simulink model "Two_Zone_MVDC_PSolver_Thermal"  (R2025b)
settings: Solver=FixedStepDiscrete  StartTime=0.0  StopTime=30  FixedStep=TsELEC  RelTol=1e-3  EnableMultiTasking=on
InitFcn:
  | TsELEC = 25e-6;
  | Ts = 25e-6;
  | TsTHERMAL = 1e-3;
  | TsCont = TsELEC;
  | Rsnub = 1e4;
undefined symbols (not defined in the file or in its folder): DiscIntNeverNeededParam, ee_sli_rtmsupport, GABDA, GABDB, GBBDA, GBBDB, gcbh, GPMMA, GPPMB, GPPMC, SADA, SADB, SADC, SADD, SBDA, SBDB, SBDC, SCDA, SCDB, SCDC, SCDD, SDDA, SDDB, SDDC, SDDD, SDDE
libraries: fl_lib x182, nesl_utility x93, ee_lib x50, SimscapeFluids_lib x4, simulink x3, slpidlib x3, eeSmAC1C x2, eePowerMeasurement x2, mcbeeMathTransformLib x2, eeTransforms x1
(part 4 of 5)

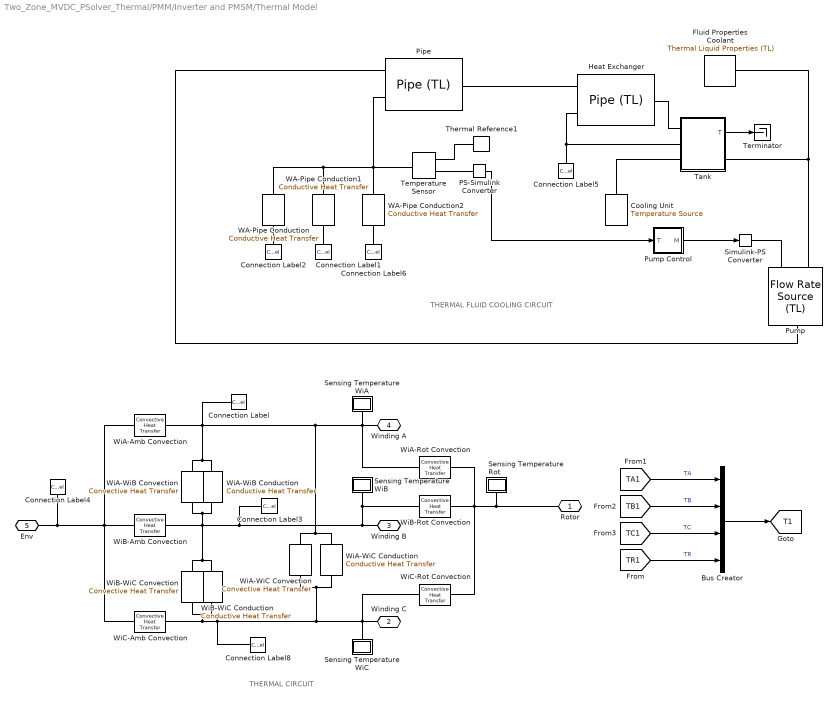
== system Two_Zone_MVDC_PSolver_Thermal/PMM/Inverter and PMSM/Thermal Model ==
  note: THERMAL CIRCUIT
  note: THERMAL FLUID COOLING CIRCUIT
  Bus Creator : BusCreator  Inputs=4
  Connection Label : ConnectionLabel  Label=WindingA
  Connection Label1 : ConnectionLabel  Label=WindingB
  Connection Label2 : ConnectionLabel  Label=WindingA
  Connection Label3 : ConnectionLabel  Label=WindingB
  Connection Label4 : ConnectionLabel  Label=Env
  Connection Label5 : ConnectionLabel  Label=Env
  Connection Label6 : ConnectionLabel  Label=WindingC
  Connection Label8 : ConnectionLabel  Label=WindingC
  Cooling Unit : fl_lib/Thermal/Thermal Sources/Temperature Source  temperature=278 K
  "Fluid Properties Coolant " : SimscapeFluids_lib/Thermal Liquid/Utilities/Thermal Liquid Properties (TL)  fluid_list=fluids.thermal_liquid.utilities.enum.thermal_liquid_fluid_list.ethylene_glycol  concentration_param_EG=fluids.thermal_liquid.utilities.enum.thermal_liquid_concentration.volume_fraction  concentration_param_PG=fluids.thermal_liquid.utilities.enum.thermal_liquid_concentration.volume_fraction  c_mass_SW=3.5e-3  c_mass_EG=0.1  c_mass_PG=0.1  c_mass_GL=0.1  c_vol_EG=0.1  c_vol_PG=0.1  beta_const_EG=2.1791 GPa  beta_const_PG=2.1791 GPa  beta_const_GL=2.1791 GPa  p_min_EG=0.01 MPa  p_min_PG=0.01 MPa  p_min_GL=0.01 MPa  p_max_EG=50 MPa  p_max_PG=50 MPa  p_max_GL=50 MPa  p_atm=0.101325 MPa  properties_range_check=simscape.enum.assert.action.error
  Heat Exchanger : SimscapeFluids_lib/Thermal Liquid/Pipes & Fittings/Pipe (TL)  dynamic_compressibility=0  inertia=0  num_segments=1  pipe_length=10 m  cross_section_geometry=fluids.thermal_liquid.pipes_fittings.enum.CrossSectionGeometry.Custom  pipe_diameter=0.1 m  pipe_inner_diameter=0.05 m  pipe_outer_diameter=0.1 m  pipe_width=0.1 m  pipe_height=0.1 m  pipe_major_axis=0.1 m  pipe_minor_axis=0.05 m  pipe_side=0.1 m  pipe_angle=30 deg  area=0.1^2/4*pi m^2  Dh=0.1128 m  elevation_spec=foundation.enum.constant_variable.constant  elevation_gain=0 m  gravity_spec=foundation.enum.constant_variable.constant  g=9.81 m/s^2  pressure_loss_spec=1  local_pressure_loss_spec=fluids.thermal_liquid.pipes_fittings.enum.LocalLossSpec.AggregateLength  length_add=0.1 m  loss_coefficient=0.1  roughness_spec=fluids.thermal_liquid.pipes_fittings.enum.RoughnessSpec.Custom  roughness=1.5e-5 m  Re_friction_TLU=[ 400 1000 1.5e+3 3e+3 4e+3 6e+3 1e+4 2e+4 4e+4 6e+4 1e+5 1e+8 ]  friction_factor_TLU=[ 0.264 0.112 0.07099999999999999 0.0417 0.0387 0.0268 0.025 0.0232 0.0226 0.022 0.0214 0.0214 ]  Re_lam=2e+3  Re_tur=4e+3  shape_factor=64  mdot_nominal=[ 0.1 1 ] kg/s  p_diff_nominal=[ 0.001 0.01 ] MPa  mdot_threshold=1e-6 kg/s  wall_spec=1  vol_expansion_spec=fluids.thermal_liquid.pipes_fittings.enum.VolumeExpansionSpec.Diameter  area_pressure_gain=1e-6 m^2/MPa  static_pressure_TLU=[.1, 1] MPa  area_pressure_gain_TLU=[1e-05, 1.1e-05] m^2  material_behavior_spec=fluids.thermal_liquid.pipes_fittings.enum.PipeMaterialBehavior.Linear  diameter_pressure_gain=1.2e-6 m/MPa  wall_thickness=0.05 m  elastic_modulus=69 GPa  stress_TLU=[276, 310] MPa  strain_TLU=[.004, .02]  stress_assert_action=simscape.enum.assert.action.none  stress_max=400 MPa  poisson_ratio=0.33  wall_time_constant=0.01 s  thermal_expansion=false  alpha_L_wall=24 um/(deltaK*m)  thermal_expansion_Tref=293.15 K  heat_transfer_spec=1  mdot_nominal_heat=[ 0.1 1 ] kg/s  T_in_nominal=[ 293.15 293.15 ] K  T_out_nominal=[ 300 300 ] K  p_in_nominal_heat=[ 0.101325 0.101325 ] MPa  T_wall_nominal=[ 303.15 303.15 ] K  a_coeff=0.023  b_Re_power=0.8  c_Pr_power=0.4  Nu_lam=3.66  Re_Colburn_TLU=[ 100 150 1000 ]  Colburn_factor_TLU=[ 0.019 0.013 0.002 ]  Re_Nu_TLU=[ 100 150 1000 ]  Pr_Nu_TLU=[ 1 10 ]  Nu_TLU=[ 3.72 4.21; 3.75 4.44; 4.21 7.15 ]  p0_vec=0.101325 MPa  T0_vec=300 K  mdot0=0.1 kg/s  p_nominal=0.101325 MPa  T_nominal=293.15 K
  PS-Simulink Converter : nesl_utility/PS-Simulink Converter  PhysicalDomain=network_engine_domain  SubClassName=ps_output  LeftPortType=input  RightPortType=output  PseudoPeriodic=off  Frequencies=[]  VectorFormat=1-D array  Unit=inherit  AffineConversion=off
  Pipe : SimscapeFluids_lib/Thermal Liquid/Pipes & Fittings/Pipe (TL)  dynamic_compressibility=0  inertia=0  num_segments=1  pipe_length=1 m  cross_section_geometry=fluids.thermal_liquid.pipes_fittings.enum.CrossSectionGeometry.Custom  pipe_diameter=0.1 m  pipe_inner_diameter=0.05 m  pipe_outer_diameter=0.1 m  pipe_width=0.1 m  pipe_height=0.1 m  pipe_major_axis=0.1 m  pipe_minor_axis=0.05 m  pipe_side=0.1 m  pipe_angle=30 deg  area=0.1^2/4*pi m^2  Dh=0.1128 m  elevation_spec=foundation.enum.constant_variable.constant  elevation_gain=0 m  gravity_spec=foundation.enum.constant_variable.constant  g=9.81 m/s^2  pressure_loss_spec=1  local_pressure_loss_spec=fluids.thermal_liquid.pipes_fittings.enum.LocalLossSpec.AggregateLength  length_add=0.1 m  loss_coefficient=0.1  roughness_spec=fluids.thermal_liquid.pipes_fittings.enum.RoughnessSpec.Custom  roughness=1.5e-5 m  Re_friction_TLU=[ 400 1000 1.5e+3 3e+3 4e+3 6e+3 1e+4 2e+4 4e+4 6e+4 1e+5 1e+8 ]  friction_factor_TLU=[ 0.264 0.112 0.07099999999999999 0.0417 0.0387 0.0268 0.025 0.0232 0.0226 0.022 0.0214 0.0214 ]  Re_lam=2e+3  Re_tur=4e+3  shape_factor=64  mdot_nominal=[ 0.1 1 ] kg/s  p_diff_nominal=[ 0.001 0.01 ] MPa  mdot_threshold=1e-6 kg/s  wall_spec=1  vol_expansion_spec=fluids.thermal_liquid.pipes_fittings.enum.VolumeExpansionSpec.Diameter  area_pressure_gain=1e-6 m^2/MPa  static_pressure_TLU=[.1, 1] MPa  area_pressure_gain_TLU=[1e-05, 1.1e-05] m^2  material_behavior_spec=fluids.thermal_liquid.pipes_fittings.enum.PipeMaterialBehavior.Linear  diameter_pressure_gain=1.2e-6 m/MPa  wall_thickness=0.05 m  elastic_modulus=69 GPa  stress_TLU=[276, 310] MPa  strain_TLU=[.004, .02]  stress_assert_action=simscape.enum.assert.action.none  stress_max=400 MPa  poisson_ratio=0.33  wall_time_constant=0.01 s  thermal_expansion=false  alpha_L_wall=24 um/(deltaK*m)  thermal_expansion_Tref=293.15 K  heat_transfer_spec=1  mdot_nominal_heat=[ 0.1 1 ] kg/s  T_in_nominal=[ 293.15 293.15 ] K  T_out_nominal=[ 300 300 ] K  p_in_nominal_heat=[ 0.101325 0.101325 ] MPa  T_wall_nominal=[ 303.15 303.15 ] K  a_coeff=0.023  b_Re_power=0.8  c_Pr_power=0.4  Nu_lam=3.66  Re_Colburn_TLU=[ 100 150 1000 ]  Colburn_factor_TLU=[ 0.019 0.013 0.002 ]  Re_Nu_TLU=[ 100 150 1000 ]  Pr_Nu_TLU=[ 1 10 ]  Nu_TLU=[ 3.72 4.21; 3.75 4.44; 4.21 7.15 ]  p0_vec=0.101325 MPa  T0_vec=300 K  mdot0=0.1 kg/s  p_nominal=0.101325 MPa  T_nominal=293.15 K
  Pump : fl_lib/Thermal Liquid/Sources/Flow Rate Source (TL)  source_type=foundation.enum.constant_controlled.controlled  flow_type=foundation.enum.mass_volumetric_flow.mass  mass_flow=0 kg/s  volumetric_flow=0 m^3/s  power_spec=foundation.enum.power_spec.isentropic  area=0.1^2/4*pi m^2
  Pump Control : Subsystem
  Sensing Temperature Rot : Subsystem
      mask Display: disp('TR')
  Sensing Temperature WiA : Subsystem
      mask Display: disp('TA')
  Sensing Temperature WiB : Subsystem
      mask Display: disp('TB')
  Sensing Temperature WiC : Subsystem
      mask Display: disp('TC')
  Simulink-PS Converter : nesl_utility/Simulink-PS Converter  PhysicalDomain=network_engine_domain  SubClassName=ps_input  LeftPortType=input  RightPortType=output  PseudoPeriodic=off  Frequencies=[]  NoiseDistribution=none  NoiseParameters=[]  Unit=1  AffineConversion=off  FilteringAndDerivatives=provide  SimscapeFilterOrder=1  InputFilterTimeConstant=0.001  UdotUserProvided=0
  Tank : Subsystem
  Temperature Sensor : fl_lib/Thermal/Thermal Sensors/Temperature Sensor  temperature_measure=foundation.enum.MeasurementReference.difference
  Terminator : Terminator
  Thermal Reference1 : fl_lib/Thermal/Thermal Elements/Thermal Reference
  WA-Pipe Conduction : fl_lib/Thermal/Thermal Elements/Conductive Heat Transfer  thermal_type=foundation.enum.ConstantVariableTabulated.Constant  wall_geometry=foundation.enum.ConductionWallGeometry.Planar  area=1 m^2  thickness=0.1 m  d_in=0.05 m  d_out=0.1 m  L=1 m  th_cond_min=10 W/(K*m)  th_cond=800 W/(m*K)  th_cond_TLU=[413, 401, 392, 383, 371, 357, 342] W/(K*m)  temp_TLU=[200, 273, 400, 600, 800, 1000, 1200] K  T_specify=off  T_priority=None  T=0 K  T_nominal_specify=off  T_nominal_value=1  T_nominal_unit=K  Q_specify=off  Q_priority=None  Q=0 J/s  Q_nominal_specify=off  Q_nominal_value=1  Q_nominal_unit=J/s
  WA-Pipe Conduction1 : fl_lib/Thermal/Thermal Elements/Conductive Heat Transfer  thermal_type=foundation.enum.ConstantVariableTabulated.Constant  wall_geometry=foundation.enum.ConductionWallGeometry.Planar  area=1 m^2  thickness=0.1 m  d_in=0.05 m  d_out=0.1 m  L=1 m  th_cond_min=10 W/(K*m)  th_cond=800 W/(m*K)  th_cond_TLU=[413, 401, 392, 383, 371, 357, 342] W/(K*m)  temp_TLU=[200, 273, 400, 600, 800, 1000, 1200] K  T_specify=off  T_priority=None  T=0 K  T_nominal_specify=off  T_nominal_value=1  T_nominal_unit=K  Q_specify=off  Q_priority=None  Q=0 J/s  Q_nominal_specify=off  Q_nominal_value=1  Q_nominal_unit=J/s
  WA-Pipe Conduction2 : fl_lib/Thermal/Thermal Elements/Conductive Heat Transfer  thermal_type=foundation.enum.ConstantVariableTabulated.Constant  wall_geometry=foundation.enum.ConductionWallGeometry.Planar  area=1 m^2  thickness=0.1 m  d_in=0.05 m  d_out=0.1 m  L=1 m  th_cond_min=10 W/(K*m)  th_cond=800 W/(m*K)  th_cond_TLU=[413, 401, 392, 383, 371, 357, 342] W/(K*m)  temp_TLU=[200, 273, 400, 600, 800, 1000, 1200] K  T_specify=off  T_priority=None  T=0 K  T_nominal_specify=off  T_nominal_value=1  T_nominal_unit=K  Q_specify=off  Q_priority=None  Q=0 J/s  Q_nominal_specify=off  Q_nominal_value=1  Q_nominal_unit=J/s
  WiA-Amb Convection : fl_lib/Thermal/Thermal Elements/Convective Heat Transfer  thermal_type=foundation.enum.constant_variable.constant  area=0.1 m^2  heat_tr_coeff=20 W/(m^2 * K)  min_heat_tr_coeff=1e-3 W/(K*m^2)  T_specify=off  T_priority=None  T=0 K  T_nominal_specify=off  T_nominal_value=1  T_nominal_unit=K  Q_specify=off  Q_priority=None  Q=0 J/s  Q_nominal_specify=off  Q_nominal_value=1  Q_nominal_unit=J/s
  WiA-Rot Convection : fl_lib/Thermal/Thermal Elements/Convective Heat Transfer  thermal_type=foundation.enum.constant_variable.constant  area=0.02 m^2  heat_tr_coeff=200 W/(m^2 * K)  min_heat_tr_coeff=1e-3 W/(K*m^2)  T_specify=off  T_priority=None  T=0 K  T_nominal_specify=off  T_nominal_value=1  T_nominal_unit=K  Q_specify=off  Q_priority=None  Q=0 J/s  Q_nominal_specify=off  Q_nominal_value=1  Q_nominal_unit=J/s
  WiA-WiB Conduction : fl_lib/Thermal/Thermal Elements/Conductive Heat Transfer  thermal_type=foundation.enum.ConstantVariableTabulated.Constant  wall_geometry=foundation.enum.ConductionWallGeometry.Planar  area=0.02 m^2  thickness=0.1 m  d_in=0.05 m  d_out=0.1 m  L=1 m  th_cond_min=10 W/(K*m)  th_cond=80 W/(m*K)  th_cond_TLU=[413, 401, 392, 383, 371, 357, 342] W/(K*m)  temp_TLU=[200, 273, 400, 600, 800, 1000, 1200] K  T_specify=off  T_priority=None  T=0 K  T_nominal_specify=off  T_nominal_value=1  T_nominal_unit=K  Q_specify=off  Q_priority=None  Q=0 J/s  Q_nominal_specify=off  Q_nominal_value=1  Q_nominal_unit=J/s
  WiA-WiB Convection : fl_lib/Thermal/Thermal Elements/Convective Heat Transfer  thermal_type=foundation.enum.constant_variable.constant  area=0.004 m^2  heat_tr_coeff=200 W/(m^2 * K)  min_heat_tr_coeff=1e-3 W/(K*m^2)  T_specify=off  T_priority=None  T=0 K  T_nominal_specify=off  T_nominal_value=1  T_nominal_unit=K  Q_specify=off  Q_priority=None  Q=0 J/s  Q_nominal_specify=off  Q_nominal_value=1  Q_nominal_unit=J/s
  WiA-WiC Conduction : fl_lib/Thermal/Thermal Elements/Conductive Heat Transfer  thermal_type=foundation.enum.ConstantVariableTabulated.Constant  wall_geometry=foundation.enum.ConductionWallGeometry.Planar  area=0.02 m^2  thickness=0.1 m  d_in=0.05 m  d_out=0.1 m  L=1 m  th_cond_min=10 W/(K*m)  th_cond=80 W/(m*K)  th_cond_TLU=[413, 401, 392, 383, 371, 357, 342] W/(K*m)  temp_TLU=[200, 273, 400, 600, 800, 1000, 1200] K  T_specify=off  T_priority=None  T=0 K  T_nominal_specify=off  T_nominal_value=1  T_nominal_unit=K  Q_specify=off  Q_priority=None  Q=0 J/s  Q_nominal_specify=off  Q_nominal_value=1  Q_nominal_unit=J/s
  WiA-WiC Convection : fl_lib/Thermal/Thermal Elements/Convective Heat Transfer  thermal_type=foundation.enum.constant_variable.constant  area=0.004 m^2  heat_tr_coeff=200 W/(m^2 * K)  min_heat_tr_coeff=1e-3 W/(K*m^2)  T_specify=off  T_priority=None  T=0 K  T_nominal_specify=off  T_nominal_value=1  T_nominal_unit=K  Q_specify=off  Q_priority=None  Q=0 J/s  Q_nominal_specify=off  Q_nominal_value=1  Q_nominal_unit=J/s
  WiB-Amb Convection : fl_lib/Thermal/Thermal Elements/Convective Heat Transfer  thermal_type=foundation.enum.constant_variable.constant  area=0.1 m^2  heat_tr_coeff=20 W/(m^2 * K)  min_heat_tr_coeff=1e-3 W/(K*m^2)  T_specify=off  T_priority=None  T=0 K  T_nominal_specify=off  T_nominal_value=1  T_nominal_unit=K  Q_specify=off  Q_priority=None  Q=0 J/s  Q_nominal_specify=off  Q_nominal_value=1  Q_nominal_unit=J/s
  WiB-Rot Convection : fl_lib/Thermal/Thermal Elements/Convective Heat Transfer  thermal_type=foundation.enum.constant_variable.constant  area=0.02 m^2  heat_tr_coeff=200 W/(m^2 * K)  min_heat_tr_coeff=1e-3 W/(K*m^2)  T_specify=off  T_priority=None  T=0 K  T_nominal_specify=off  T_nominal_value=1  T_nominal_unit=K  Q_specify=off  Q_priority=None  Q=0 J/s  Q_nominal_specify=off  Q_nominal_value=1  Q_nominal_unit=J/s
  WiB-WiC Conduction : fl_lib/Thermal/Thermal Elements/Conductive Heat Transfer  thermal_type=foundation.enum.ConstantVariableTabulated.Constant  wall_geometry=foundation.enum.ConductionWallGeometry.Planar  area=0.02 m^2  thickness=0.1 m  d_in=0.05 m  d_out=0.1 m  L=1 m  th_cond_min=10 W/(K*m)  th_cond=80 W/(m*K)  th_cond_TLU=[413, 401, 392, 383, 371, 357, 342] W/(K*m)  temp_TLU=[200, 273, 400, 600, 800, 1000, 1200] K  T_specify=off  T_priority=None  T=0 K  T_nominal_specify=off  T_nominal_value=1  T_nominal_unit=K  Q_specify=off  Q_priority=None  Q=0 J/s  Q_nominal_specify=off  Q_nominal_value=1  Q_nominal_unit=J/s
  WiB-WiC Convection : fl_lib/Thermal/Thermal Elements/Convective Heat Transfer  thermal_type=foundation.enum.constant_variable.constant  area=0.004 m^2  heat_tr_coeff=200 W/(m^2 * K)  min_heat_tr_coeff=1e-3 W/(K*m^2)  T_specify=off  T_priority=None  T=0 K  T_nominal_specify=off  T_nominal_value=1  T_nominal_unit=K  Q_specify=off  Q_priority=None  Q=0 J/s  Q_nominal_specify=off  Q_nominal_value=1  Q_nominal_unit=J/s
  WiC-Amb Convection : fl_lib/Thermal/Thermal Elements/Convective Heat Transfer  thermal_type=foundation.enum.constant_variable.constant  area=0.05 m^2  heat_tr_coeff=20 W/(m^2 * K)  min_heat_tr_coeff=1e-3 W/(K*m^2)  T_specify=off  T_priority=None  T=0 K  T_nominal_specify=off  T_nominal_value=1  T_nominal_unit=K  Q_specify=off  Q_priority=None  Q=0 J/s  Q_nominal_specify=off  Q_nominal_value=1  Q_nominal_unit=J/s
  WiC-Rot Convection : fl_lib/Thermal/Thermal Elements/Convective Heat Transfer  thermal_type=foundation.enum.constant_variable.constant  area=0.02 m^2  heat_tr_coeff=200 W/(m^2 * K)  min_heat_tr_coeff=1e-3 W/(K*m^2)  T_specify=off  T_priority=None  T=0 K  T_nominal_specify=off  T_nominal_value=1  T_nominal_unit=K  Q_specify=off  Q_priority=None  Q=0 J/s  Q_nominal_specify=off  Q_nominal_value=1  Q_nominal_unit=J/s
  Rotor : PMIOPort  Side=Left
  Winding C : PMIOPort  Port=2  Side=Right
  Winding B : PMIOPort  Port=3  Side=Right
  Winding A : PMIOPort  Port=4  Side=Right
  Env : PMIOPort  Port=5  Side=Left
  tag scope: T1=global
  wires:
  Bus Creator/1 -> [T1]
  PS-Simulink Converter/1 -> Pump Control/1(T)
  Tank/1(T) -> Terminator/1
  [TA1] -> Bus Creator/1  "TA"
  [TB1] -> Bus Creator/2  "TB"
  [TC1] -> Bus Creator/3  "TC"
  [TR1] -> Bus Creator/4  "TR"
  Pump Control/1(M) -> Simulink-PS Converter/1
  connections:
  WiB-Amb Convection/RConn1 -- Connection Label4/LConn1 -- Env/RConn1 -- WiC-Amb Convection/RConn1 -- WiA-Amb Convection/RConn1
  Sensing Temperature WiC/LConn1 -- WiA-WiC Conduction/LConn1 -- WiA-WiC Convection/LConn1 -- Connection Label8/LConn1 -- WiC-Amb Convection/LConn1 -- WiB-WiC Convection/RConn1 -- WiB-WiC Conduction/RConn1 -- Winding C/RConn1 -- WiC-Rot Convection/RConn1
  WiB-WiC Convection/LConn1 -- WiB-WiC Conduction/LConn1 -- Connection Label3/LConn1 -- Winding B/RConn1 -- WiB-Rot Convection/RConn1 -- Sensing Temperature WiB/LConn1 -- WiB-Amb Convection/LConn1 -- WiA-WiB Conduction/RConn1 -- WiA-WiB Convection/RConn1
  Winding A/RConn1 -- Sensing Temperature WiA/LConn1 -- Connection Label/LConn1 -- WiA-Amb Convection/LConn1 -- WiA-WiB Conduction/LConn1 -- WiA-WiB Convection/LConn1 -- WiA-WiC Convection/RConn1 -- WiA-WiC Conduction/RConn1 -- WiA-Rot Convection/RConn1
  Tank/RConn1 -- "Fluid Properties Coolant "/RConn1 -- Pump/LConn1
  WiA-Rot Convection/LConn1 -- WiB-Rot Convection/LConn1 -- WiC-Rot Convection/LConn1 -- Rotor/RConn1 -- Sensing Temperature Rot/LConn1
  PS-Simulink Converter/LConn1 -- Temperature Sensor/RConn2
  Simulink-PS Converter/RConn1 -- Pump/LConn2
  Tank/LConn1 -- Heat Exchanger/RConn1
  Heat Exchanger/LConn1 -- Pipe/RConn1
  Tank/LConn3 -- Cooling Unit/LConn1
  Thermal Reference1/LConn1 -- Temperature Sensor/RConn1
  Pipe/LConn1 -- Pump/RConn1
  Temperature Sensor/LConn1 -- WA-Pipe Conduction2/RConn1 -- WA-Pipe Conduction1/RConn1 -- WA-Pipe Conduction/RConn1 -- Pipe/LConn2
  Tank/LConn2 -- Heat Exchanger/LConn2 -- Connection Label5/LConn1
  WA-Pipe Conduction/LConn1 -- Connection Label2/LConn1
  WA-Pipe Conduction1/LConn1 -- Connection Label1/LConn1
  WA-Pipe Conduction2/LConn1 -- Connection Label6/LConn1

== system Two_Zone_MVDC_PSolver_Thermal/PMM/Inverter and PMSM/measVI ==
  Current Sensor (Three-Phase) : ee_lib/Sensors & Transducers/Current Sensor (Three-Phase)
  Line Voltage Sensor (Three-Phase) : ee_lib/Sensors & Transducers/Line Voltage Sensor (Three-Phase)
  PS-Simulink Converter2 : nesl_utility/PS-Simulink Converter  PhysicalDomain=network_engine_domain  SubClassName=ps_output  LeftPortType=input  RightPortType=output  PseudoPeriodic=off  Frequencies=[]  VectorFormat=1-D array  Unit=inherit  AffineConversion=off
  PS-Simulink Converter3 : nesl_utility/PS-Simulink Converter  PhysicalDomain=network_engine_domain  SubClassName=ps_output  LeftPortType=input  RightPortType=output  PseudoPeriodic=off  Frequencies=[]  VectorFormat=1-D array  Unit=inherit  AffineConversion=off
  ~1 : PMIOPort  Side=Left
  ~2 : PMIOPort  Port=2  Side=Right
  tag scope: Iabc1=global, Vabc1=global
  wires:
  PS-Simulink Converter3/1 -> [Iabc1]  "Iabc 1"
  PS-Simulink Converter2/1 -> [Vabc1]  "Vabc 1"
  connections:
  Current Sensor (Three-Phase)/LConn1 -- ~1/RConn1 -- Line Voltage Sensor (Three-Phase)/LConn1
  Current Sensor (Three-Phase)/RConn2 -- ~2/RConn1
  PS-Simulink Converter2/LConn1 -- Line Voltage Sensor (Three-Phase)/RConn1
  Current Sensor (Three-Phase)/RConn1 -- PS-Simulink Converter3/LConn1

== system Two_Zone_MVDC_PSolver_Thermal/PMM/Speed Reference/LPF ==
  u : Inport
  Discrete-Time Integrator : DiscreteIntegrator  gainval=20  SampleTime=TsELEC  ICPrevOutput=DiscIntNeverNeededParam  ICPrevScaledInput=DiscIntNeverNeededParam
  Sum : Sum  Inputs=|+-
  y : Outport
  wires:
  u/1 -> Sum/1
  Discrete-Time Integrator/1 -> Sum/2, y/1
  Sum/1 -> Discrete-Time Integrator/1

== system Two_Zone_MVDC_PSolver_Thermal/PGM1/Gas turbine/Turbine and governor /Gas Turbine ==
  1/T_GT : fl_lib/Physical Signals/Functions/PS Gain  gain=1/T_GT 1/s
  PS Integrator : fl_lib/Physical Signals/Linear Operators/PS Integrator  reset_method=foundation.enum.IntegratorResetSpec.None  initial_condition_spec=foundation.enum.IntegratorICSpec.Internal  saturation_spec=foundation.enum.IntegratorSaturationSpec.None  saturation_source_spec=foundation.enum.IntegratorSaturationSourceSpec.Internal  x0=pu_torque0 s  xu=inf s  xl=-inf s
  PS Subtract1 : fl_lib/Physical Signals/Functions/PS Subtract
  delta_y : PMIOPort  Side=Left
  torque : PMIOPort  Port=2  Side=Right
  connections:
  torque/RConn1 -- PS Subtract1/LConn2 -- PS Integrator/RConn1
  PS Subtract1/RConn1 -- 1/T_GT/LConn1
  PS Subtract1/LConn1 -- delta_y/RConn1
  1/T_GT/RConn1 -- PS Integrator/LConn1

== system Two_Zone_MVDC_PSolver_Thermal/PGM1/Gas turbine/Turbine and governor /Governor ==
  1 : fl_lib/Physical Signals/Functions/PS Gain  gain=1 1/s
  1/T_G : fl_lib/Physical Signals/Functions/PS Gain  gain=1/T_G
  1/droop : fl_lib/Physical Signals/Functions/PS Gain  gain=1/(droop_percentage/100)
  Delta load setpoint : fl_lib/Physical Signals/Functions/PS Subtract
  Delta speed : fl_lib/Physical Signals/Functions/PS Subtract
  Load_setpoint : fl_lib/Physical Signals/Sources/PS Constant  constant=pu_load_reference_setpoint
  PS Integrator : fl_lib/Physical Signals/Linear Operators/PS Integrator  reset_method=foundation.enum.IntegratorResetSpec.None  initial_condition_spec=foundation.enum.IntegratorICSpec.Internal  saturation_spec=foundation.enum.IntegratorSaturationSpec.None  saturation_source_spec=foundation.enum.IntegratorSaturationSourceSpec.Internal  x0=pu_torque0 s  xu=inf s  xl=-inf s
  PS Subtract1 : fl_lib/Physical Signals/Functions/PS Subtract
  Rotor Velocity Measurement : ee_lib/Electromechanical/Synchronous/Synchronous Machine Measurement  output_idx=4
      settings: InternalSimscapePortConfiguration="{\"Bottom\":[],\"Left\":[{\"id\":\"pu_input\",\"label\":\"pu\",\"type\":\"input\"}],\"Right\":[{\"id\":\"pu_output\",\"label\":\"o\",\"type\":\"output\"}],\"Top\":[]}"
  Speed_ref : fl_lib/Physical Signals/Sources/PS Constant  constant=pu_speed_reference
  pu : PMIOPort  Side=Left
  delta_y : PMIOPort  Port=2  Side=Right
  connections:
  pu/RConn1 -- Rotor Velocity Measurement/LConn1
  Delta load setpoint/RConn1 -- PS Subtract1/LConn1
  Delta load setpoint/LConn2 -- 1/droop/RConn1
  Rotor Velocity Measurement/RConn1 -- Delta speed/LConn1
  Speed_ref/RConn1 -- Delta speed/LConn2
  1/droop/LConn1 -- Delta speed/RConn1
  Load_setpoint/RConn1 -- Delta load setpoint/LConn1
  1/T_G/RConn1 -- PS Integrator/LConn1
  PS Subtract1/RConn1 -- 1/T_G/LConn1
  1/RConn1 -- PS Subtract1/LConn2
  PS Integrator/RConn1 -- delta_y/RConn1 -- 1/LConn1

== system Two_Zone_MVDC_PSolver_Thermal/PGM2/Gas turbine/Turbine and governor /Gas Turbine ==
  1/T_GT : fl_lib/Physical Signals/Functions/PS Gain  gain=1/T_GT 1/s
  PS Integrator : fl_lib/Physical Signals/Linear Operators/PS Integrator  reset_method=foundation.enum.IntegratorResetSpec.None  initial_condition_spec=foundation.enum.IntegratorICSpec.Internal  saturation_spec=foundation.enum.IntegratorSaturationSpec.None  saturation_source_spec=foundation.enum.IntegratorSaturationSourceSpec.Internal  x0=pu_torque0 s  xu=inf s  xl=-inf s
  PS Subtract1 : fl_lib/Physical Signals/Functions/PS Subtract
  delta_y : PMIOPort  Side=Left
  torque : PMIOPort  Port=2  Side=Right
  connections:
  torque/RConn1 -- PS Subtract1/LConn2 -- PS Integrator/RConn1
  PS Subtract1/RConn1 -- 1/T_GT/LConn1
  PS Subtract1/LConn1 -- delta_y/RConn1
  1/T_GT/RConn1 -- PS Integrator/LConn1

== system Two_Zone_MVDC_PSolver_Thermal/PGM2/Gas turbine/Turbine and governor /Governor ==
  1 : fl_lib/Physical Signals/Functions/PS Gain  gain=1 1/s
  1/T_G : fl_lib/Physical Signals/Functions/PS Gain  gain=1/T_G
  1/droop : fl_lib/Physical Signals/Functions/PS Gain  gain=1/(droop_percentage/100)
  Delta load setpoint : fl_lib/Physical Signals/Functions/PS Subtract
  Delta speed : fl_lib/Physical Signals/Functions/PS Subtract
  Load_setpoint : fl_lib/Physical Signals/Sources/PS Constant  constant=pu_load_reference_setpoint
  PS Integrator : fl_lib/Physical Signals/Linear Operators/PS Integrator  reset_method=foundation.enum.IntegratorResetSpec.None  initial_condition_spec=foundation.enum.IntegratorICSpec.Internal  saturation_spec=foundation.enum.IntegratorSaturationSpec.None  saturation_source_spec=foundation.enum.IntegratorSaturationSourceSpec.Internal  x0=pu_torque0 s  xu=inf s  xl=-inf s
  PS Subtract1 : fl_lib/Physical Signals/Functions/PS Subtract
  Rotor Velocity Measurement : ee_lib/Electromechanical/Synchronous/Synchronous Machine Measurement  output_idx=4
      settings: InternalSimscapePortConfiguration="{\"Bottom\":[],\"Left\":[{\"id\":\"pu_input\",\"label\":\"pu\",\"type\":\"input\"}],\"Right\":[{\"id\":\"pu_output\",\"label\":\"o\",\"type\":\"output\"}],\"Top\":[]}"
  Speed_ref : fl_lib/Physical Signals/Sources/PS Constant  constant=pu_speed_reference
  pu : PMIOPort  Side=Left
  delta_y : PMIOPort  Port=2  Side=Right
  connections:
  pu/RConn1 -- Rotor Velocity Measurement/LConn1
  Delta load setpoint/RConn1 -- PS Subtract1/LConn1
  Delta load setpoint/LConn2 -- 1/droop/RConn1
  Rotor Velocity Measurement/RConn1 -- Delta speed/LConn1
  Speed_ref/RConn1 -- Delta speed/LConn2
  1/droop/LConn1 -- Delta speed/RConn1
  Load_setpoint/RConn1 -- Delta load setpoint/LConn1
  1/T_G/RConn1 -- PS Integrator/LConn1
  PS Subtract1/RConn1 -- 1/T_G/LConn1
  1/RConn1 -- PS Subtract1/LConn2
  PS Integrator/RConn1 -- 1/LConn1 -- delta_y/RConn1

== system Two_Zone_MVDC_PSolver_Thermal/PMM/Control/Speed Control/PI_Controller_Speed ==
  N_ref : Inport
  N_fb : Inport  Port=2
  Constant : Constant  Value=0  SampleTime=TsELEC
  Discrete PID Controller : slpidlib/PID Controller  Controller=PID  Form=Parallel  TimeDomain=Discrete-time  UseExternalTs=off  SampleTime=TsELEC  IntegratorMethod=Forward Euler  FilterMethod=Forward Euler  ControllerParametersSource=internal  P=500  I=200*10  UseKiTs=off  D=0  UseExternalDerivativeSource=off  N=100  UseFilter=on  TunerSelectOption=Transfer Function Based (PID Tuner App)  InitialConditionSource=internal  InitialConditionForIntegrator=0  InitialConditionForFilter=0  DifferentiatorICPrevScaledInput=0  ExternalReset=either  TrackingMode=off  Kt=1  LimitOutput=off  SatLimitsSource=internal  UpperSaturationLimit=inf  LowerSaturationLimit=-inf  LinearizeAsGain=off  AntiWindupMode=none  Kb=1  LimitIntegrator=off  UpperIntegratorSaturationLimit=inf  LowerIntegratorSaturationLimit=-inf  POutMin=[]  POutMax=[]  IOutMin=[]  IOutMax=[]  DOutMin=[]  DOutMax=[]  NOutMin=[]  NOutMax=[]  SumOutMin=[]  SumOutMax=[]  SaturationOutMin=[]  SaturationOutMax=[]  PParamMin=[]  PParamMax=[]  IParamMin=[]  IParamMax=[]  DParamMin=[]  DParamMax=[]  NParamMin=[]  NParamMax=[]  KbParamMin=[]  KbParamMax=[]  KtParamMin=[]  KtParamMax=[]  KbOutMin=[]  KbOutMax=[]  KtOutMin=[]  KtOutMax=[]  IntegratorOutMin=[]  IntegratorOutMax=[]  FilterOutMin=[]  FilterOutMax=[]  SumI1OutMin=[]  SumI1OutMax=[]  SumI2OutMin=[]  SumI2OutMax=[]  SumI3OutMin=[]  SumI3OutMax=[]  SumI4OutMin=[]  SumI4OutMax=[]  SumDOutMin=[]  SumDOutMax=[]  DifferentiatorOutMin=[]  DifferentiatorOutMax=[]  FilterDiffOutCoefMin=[]  FilterDiffOutCoefMax=[]  ReciprocalOutMin=[]  ReciprocalOutMax=[]  SumDenOutMin=[]  SumDenOutMax=[]  SumNumOutMin=[]  SumNumOutMax=[]  DivideOutMin=[]  DivideOutMax=[]  UdiffTsProdOutMin=[]  UdiffTsProdOutMax=[]  NTsProdOutMin=[]  NTsProdOutMax=[]  UintegralTsProdOutMin=[]  UintegralTsProdOutMax=[]  UngainTsProdOutMin=[]  UngainTsProdOutMax=[]  ClampingZeroOutDataTypeStr=Inherit: Inherit via back propagation  ClampingZeroOutMin=[]  ClampingZeroOutMax=[]  FilterDenConstantOutDataTypeStr=Inherit: Inherit via back propagation  FilterDenConstantOutMin=[]  FilterDenConstantOutMax=[]  PCopyOutDataTypeStr=Inherit: Inherit via back propagation  PCopyOutMin=[]  PCopyOutMax=[]  NCopyOutDataTypeStr=Inherit: Inherit via back propagation  NCopyOutMin=[]  NCopyOutMax=[]  IntegratorContinuousStateAttributes=''  IntegratorStateMustResolveToSignalObject=off  IntegratorRTWStateStorageClass=Auto  FilterContinuousStateAttributes=''  FilterStateMustResolveToSignalObject=off  FilterRTWStateStorageClass=Auto  ParallelPVariant=InternalParameters  IdealPVariant=Disabled  IVariant=InternalParameters  DVariant=InternalParameters  IntegratorVariant=Discrete  SatVariant=Disabled  AWVariant=Passthrough  PCopyVariant=Disabled  TRVariant=Disabled  FdbkBlocksVariant=Forward  IdealPFdbkVariant=Disabled  SatFdbkVariant=Disabled  DerivativeFilterVariant=ForwardEulerFilter  NVariant=InternalParameters  NCopyVariant=Disabled  FilterICVariant=InternalICsFilter  IntegratorICVariant=InternalICs  ExternalResetVariant=ExternalReset  TRSumVariant=Passthrough  SumFdbkVariant=Disabled  SumVariant=Sum_PID  TsampFilterVariant=InternalTs  TsampNgainVariant=Passthrough  TsampIntegralVariant=Disabled_SignalSpec  ExternalSaturationOutDataTypeStr=Inherit: Same as second input  DerivativeSourceVariant=ErrorSignal  PreIntVariant=InternalPreInt
  Sum : Sum  Inputs=|+-  RndMeth=Round
  Iq_ref : Outport  VectorParamsAs1DForOutWhenUnconnected=off
  wires:
  N_fb/1 -> Sum/2
  N_ref/1 -> Sum/1
  Sum/1 -> Discrete PID Controller/1
  Discrete PID Controller/1 -> Iq_ref/1
  Constant/1 -> Discrete PID Controller/2

== system Two_Zone_MVDC_PSolver_Thermal/PMM/Control/Torque Control/Control_System ==
  Iab_meas_PU : Inport
  Pos_PU : Inport  Port=2
  Idq_ref_PU : Inport  Port=3
  Clarke Transform : mcbeeMathTransformLib/Clarke Transform  PowerInvariant=off  UseWithEmbedded=off  PhaseInput=Two inputs
  Clarke to Park Angle Transform : mcbeeMathTransformLib/Clarke to Park Angle Transform  AxisAlignment=D-axis  UseWithEmbedded=off  PhaseInput=Two inputs  ThetaInput=Sine and Cosine electrical position  AngleInput=Per-unit  N_points=1024
  Constant : Constant  Value=0  SampleTime=TsELEC
  Constant1 : Constant  Value=sqrt(3)  SampleTime=TsELEC
  Current_Controllers : Subsystem
  Demux1 : Demux  Outputs=3
  Inverse Park Transform : eeTransforms/Inverse Park Transform  AxisAlignment=D-axis  PowerInvariant=off
  Mux : Mux  Inputs=3
  "PWM Generator (Three-phase, Two-level)" : Subsystem  LoadFcn=ee_sli_rtmsupport( 'loadfcn', gcbh );  mask(PWM Generator (three-phase, two-level)){PWMMode=Continuous PWM (CPWM), CPWMMode=SVM: space vector modulation, DPWMMode=60 DPWM: 60 degree discontinuous PWM, SamplingMode=Natural, fsw=1/TsELEC/10, Ts=TsELEC}
      mask prompts: PWMMode "physmod:ee:library:comments:control:eePwmGeneratorTwoLevel:PWMMode_MP"; CPWMMode "physmod:ee:library:comments:control:eePwmGeneratorTwoLevel:ContinuousPWM_MP"; DPWMMode "physmod:ee:library:comments:control:eePwmGeneratorTwoLevel:DiscontinuousPWM_MP"; SamplingMode "physmod:ee:library:comments:control:eePwmGeneratorTwoLevel:SamplingMode_MP"; fsw "physmod:ee:library:comments:control:eePwmGeneratorTwoLevel:SwitchingFrequencyHz_MP"; Ts "physmod:ee:library:comments:control:eePwmGeneratorTwoLevel:SampleTimes_MP"
      mask help: physmod:ee:library:comments:control:eePwmGeneratorTwoLevel:PWMGeneratorthreephaseTwolevel_MD
      mask init:
      | Tsw = 1/fsw;
      | 
      | if fsw <= 0
      |     error(message('physmod:simscape:compiler:patterns:checks:GreaterThanZero',getString(message('physmod:ee:library:comments:control:eePwmGeneratorTwoLevel:SwitchingFrequencyHz_MP'))));
      | end
      | 
      | if Ts <= 0
      |     error(message('physmod:simscape:compiler:patterns:checks:GreaterThanZero',getString(message('physmod:ee:library:comments:control:eePwmGeneratorTwoLevel:SampleTimes_MP'))));
      | end
      | 
      | if Ts > 1/(10*fsw)
      |     error(message('physmod:simscape:compiler:patterns:checks:LessThanOrEqual',getString(message('physmod:ee:library:comments:control:eePwmGeneratorTwoLevel:SampleTimes_MP')),getString(message('physmod:ee:library:comments:control:eePwmGeneratorTwoLevel:inverseOf10TimesSwitchingFrequency_MP'))));
      | end
      | 
      | switch SamplingMode
      |     case 'Natural'
      |         RateTransitionOnInput = -1;
      |         GateGeneratorX0 = 0;
      |     case 'Asymmetric'
      |         RateTransitionOnInput = 0.5*Tsw;
      |         GateGeneratorX0 = 0.5/fsw;
      |     case 'Symmetric'
      |         RateTransitionOnInput = Tsw;
      |         GateGeneratorX0 = 0;
      | end
      | 
      | 
      | switch PWMMode
      |     case 'Continuous PWM (CPWM)'
      |         switch CPWMMode
      |             case 'SPWM: sinusoidal PWM'
      |                 PWM = 1;
      |             case 'SVM: space vector modulation'
      |                 PWM = 2;
      |         end
      |     case 'Discontinuous PWM (DPWM)'
      |         switch DPWMMode
      |             case '60 DPWM: 60 degree discontinuous PWM'
      |                 PWM = 3;
      |             case '60 DPWM (+30 degree shift): +30 degree shift from 60 DPWM'
      |                 PWM = 4;
      |             case '60 DPWM (-30 degree shift): -30 degree shift from 60 DPWM'
      |                 PWM = 5;
      |             case '30 DPWM: 30 degree discontinuous PWM'
      |                 PWM = 6;
      |             case '120 DPWM: positive dc component'
      |                 PWM = 7;
      |             case '120 DPWM: negative dc component'
      |                 PWM = 8;
      |         end
      | end
      settings: CopyFcn=ee_sli_rtmsupport( 'copyfcn', gcbh );  DeleteFcn=ee_sli_rtmsupport( 'deletefcn', gcbh );  ModelCloseFcn=ee_sli_rtmsupport( 'modelclosefcn', gcbh );  PreSaveFcn=%pe_sli_rtmsupport( 'presavefcn', gcbh );  PostSaveFcn=ee_sli_rtmsupport( 'postsavefcn', gcbh );  PreCopyFcn=ee_sli_rtmsupport( 'precopyfcn', gcbh );  OpenFcn=ee_sli_rtmsupport( 'openfcn', gcbh );  CloseFcn=ee_sli_rtmsupport( 'closefcn', gcbh );  PreDeleteFcn=ee_sli_rtmsupport( 'predeletefcn', gcbh );
      mask Help: web(nesl_help(gcbh))
      mask TypeOptions PWMMode: physmod:ee:library:comments:control:eePwmGeneratorTwoLevel:ContinuousPWMCPWM_PV | physmod:ee:library:comments:control:eePwmGeneratorTwoLevel:DiscontinuousPWMDPWM_PV
      mask Callback PWMMode:
      | switch get_param(gcb,'PWMMode')
      |     case 'Continuous PWM (CPWM)'
      |         set_param(gcb,'MaskVisibilities',{'on';'on';'off';'on';'on';'on'})
      |     case 'Discontinuous PWM (DPWM)'
      |         set_param(gcb,'MaskVisibilities',{'on';'off';'on';'on';'on';'on'})
      | end
      mask TypeOptions CPWMMode: physmod:ee:library:comments:control:eePwmGeneratorTwoLevel:SPWMSinusoidalPWM_PV | physmod:ee:library:comments:control:eePwmGeneratorTwoLevel:SVMSpaceVectorModulation_PV
      mask TypeOptions DPWMMode: physmod:ee:library:comments:control:eePwmGeneratorTwoLevel:x60DPWM60DegreeDiscontinuousPWM_PV | physmod:ee:library:comments:control:eePwmGeneratorTwoLevel:x60DPWM30DegreeShift30DegreeShiftFrom60DPWM_PV | physmod:ee:library:comments:control:eePwmGeneratorTwoLevel:x60DPWM0x2D30DegreeShift0x2D30DegreeShiftFrom60DPWM_PV | physmod:ee:library:comments:control:eePwmGeneratorTwoLevel:x30DPWM30DegreeDiscontinuousPWM_PV | physmod:ee:library:comments:control:eePwmGeneratorTwoLevel:x120DPWMPositiveDcComponent_PV | physmod:ee:library:comments:control:eePwmGeneratorTwoLevel:x120DPWMNegativeDcComponent_PV
      mask TypeOptions SamplingMode: physmod:ee:library:comments:control:eePwmGeneratorTwoLevel:Natural_PV | physmod:ee:library:comments:control:eePwmGeneratorTwoLevel:Asymmetric_PV | physmod:ee:library:comments:control:eePwmGeneratorTwoLevel:Symmetric_PV
      mask DialogControl ParameterGroupVar Prompt: physmod:ee:library:comments:control:eePwmGeneratorTwoLevel:tab_Parameters
      mask DialogControl PWMMode Prompt: PWM mode
      mask DialogControl CPWMMode Prompt: Continuous PWM
      mask DialogControl DPWMMode Prompt: Discontinuous PWM
      mask DialogControl SamplingMode Prompt: Sampling mode
      mask DialogControl fsw Prompt: Switching frequency (Hz)
      mask DialogControl Ts Prompt: Sample time (s)
  Terminator : Terminator
  Terminator1 : Terminator
  ab2abc : Subsystem
  Vabc in PU : Outport  VectorParamsAs1DForOutWhenUnconnected=off
  wires:
  Idq_ref_PU/1 -> Current_Controllers/3(Idq_ref_PU)
  Clarke Transform/1 -> Clarke to Park Angle Transform/1
  Iab_meas_PU/1 -> ab2abc/1(ab)
  ab2abc/1(abc) -> Clarke Transform/1
  Clarke to Park Angle Transform/1 -> Demux1/1
  Demux1/1 -> Current_Controllers/1(Id)
  Demux1/2 -> Current_Controllers/2(Iq)
  Demux1/3 -> Terminator1/1
  Current_Controllers/1(Vd_ref) -> Mux/1
  Pos_PU/1 -> Inverse Park Transform/2, Clarke to Park Angle Transform/2
  Current_Controllers/2(Vq_ref) -> Mux/2
  Constant/1 -> Mux/3
  Constant1/1 -> "PWM Generator (Three-phase, Two-level)"/2(vdc)
  "PWM Generator (Three-phase, Two-level)"/1(g) -> Terminator/1
  "PWM Generator (Three-phase, Two-level)"/2(ModWave) -> Vabc in PU/1  "ModWave"
  Mux/1 -> Inverse Park Transform/1
  Inverse Park Transform/1 -> "PWM Generator (Three-phase, Two-level)"/1(Vabc)

== system Two_Zone_MVDC_PSolver_Thermal/PMM/Inverter and PMSM/Thermal Model/Pump Control ==
  T : Inport
  Discrete-Time Integrator : DiscreteIntegrator  gainval=10  SampleTime=-1  ICPrevOutput=DiscIntNeverNeededParam  ICPrevScaledInput=DiscIntNeverNeededParam
  Gain : Gain  Gain=100
  Relay : Relay  OnSwitchValue=329  OffSwitchValue=320  ZeroCross=off
  Sum : Sum  Inputs=|+-
  M : Outport  VectorParamsAs1DForOutWhenUnconnected=off
  wires:
  Gain/1 -> M/1  "pump"
  Sum/1 -> Discrete-Time Integrator/1
  Relay/1 -> Sum/1  "Pump_flw"
  T/1 -> Relay/1
  Discrete-Time Integrator/1 -> Gain/1, Sum/2

== system Two_Zone_MVDC_PSolver_Thermal/PMM/Inverter and PMSM/Thermal Model/Sensing Temperature Rot ==
  PS-Simulink Converter : nesl_utility/PS-Simulink Converter  PhysicalDomain=network_engine_domain  SubClassName=ps_output  LeftPortType=input  RightPortType=output  PseudoPeriodic=off  Frequencies=[]  VectorFormat=1-D array  Unit=degC  AffineConversion=on
  Temperature Sensor : fl_lib/Thermal/Thermal Sensors/Temperature Sensor  temperature_measure=foundation.enum.MeasurementReference.difference
  ThRef : fl_lib/Thermal/Thermal Elements/Thermal Reference
  H : PMIOPort  Side=Left
  tag scope: TR1=global
  wires:
  PS-Simulink Converter/1 -> [TR1]
  connections:
  H/RConn1 -- Temperature Sensor/LConn1
  ThRef/LConn1 -- Temperature Sensor/RConn1
  Temperature Sensor/RConn2 -- PS-Simulink Converter/LConn1

== system Two_Zone_MVDC_PSolver_Thermal/PMM/Inverter and PMSM/Thermal Model/Sensing Temperature WiA ==
  PS-Simulink Converter : nesl_utility/PS-Simulink Converter  PhysicalDomain=network_engine_domain  SubClassName=ps_output  LeftPortType=input  RightPortType=output  PseudoPeriodic=off  Frequencies=[]  VectorFormat=1-D array  Unit=degC  AffineConversion=on
  Temperature Sensor : fl_lib/Thermal/Thermal Sensors/Temperature Sensor  temperature_measure=foundation.enum.MeasurementReference.difference
  ThRef : fl_lib/Thermal/Thermal Elements/Thermal Reference
  H : PMIOPort  Side=Left
  tag scope: TA1=global
  wires:
  PS-Simulink Converter/1 -> [TA1]
  connections:
  Temperature Sensor/RConn2 -- PS-Simulink Converter/LConn1
  ThRef/LConn1 -- Temperature Sensor/RConn1
  H/RConn1 -- Temperature Sensor/LConn1

== system Two_Zone_MVDC_PSolver_Thermal/PMM/Inverter and PMSM/Thermal Model/Sensing Temperature WiB ==
  PS-Simulink Converter : nesl_utility/PS-Simulink Converter  PhysicalDomain=network_engine_domain  SubClassName=ps_output  LeftPortType=input  RightPortType=output  PseudoPeriodic=off  Frequencies=[]  VectorFormat=1-D array  Unit=degC  AffineConversion=on
  Temperature Sensor : fl_lib/Thermal/Thermal Sensors/Temperature Sensor  temperature_measure=foundation.enum.MeasurementReference.difference
  ThRef : fl_lib/Thermal/Thermal Elements/Thermal Reference
  H : PMIOPort  Side=Left
  tag scope: TB1=global
  wires:
  PS-Simulink Converter/1 -> [TB1]
  connections:
  H/RConn1 -- Temperature Sensor/LConn1
  ThRef/LConn1 -- Temperature Sensor/RConn1
  Temperature Sensor/RConn2 -- PS-Simulink Converter/LConn1

== system Two_Zone_MVDC_PSolver_Thermal/PMM/Inverter and PMSM/Thermal Model/Sensing Temperature WiC ==
  PS-Simulink Converter : nesl_utility/PS-Simulink Converter  PhysicalDomain=network_engine_domain  SubClassName=ps_output  LeftPortType=input  RightPortType=output  PseudoPeriodic=off  Frequencies=[]  VectorFormat=1-D array  Unit=degC  AffineConversion=on
  Temperature Sensor : fl_lib/Thermal/Thermal Sensors/Temperature Sensor  temperature_measure=foundation.enum.MeasurementReference.difference
  ThRef : fl_lib/Thermal/Thermal Elements/Thermal Reference
  H : PMIOPort  Side=Left
  tag scope: TC1=global
  wires:
  PS-Simulink Converter/1 -> [TC1]
  connections:
  Temperature Sensor/RConn2 -- PS-Simulink Converter/LConn1
  ThRef/LConn1 -- Temperature Sensor/RConn1
  H/RConn1 -- Temperature Sensor/LConn1

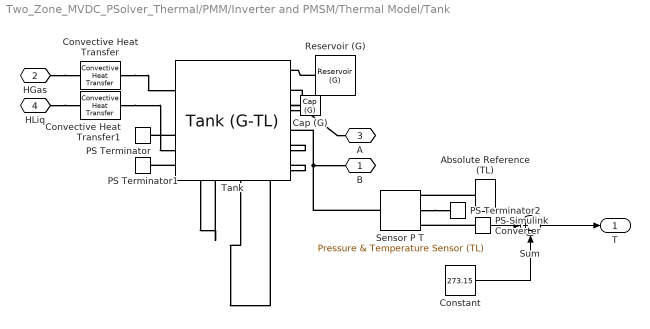
== system Two_Zone_MVDC_PSolver_Thermal/PMM/Inverter and PMSM/Thermal Model/Tank ==
  Absolute Reference (TL) : fl_lib/Thermal Liquid/Elements/Absolute Reference (TL)
  Cap (G) : fl_lib/Gas/Elements/Cap (G)  p_specify=off  p_priority=None  p=0.101325 MPa  p_nominal_specify=off  p_nominal_value=1  p_nominal_unit=MPa  T_specify=off  T_priority=None  T=293.15 K  T_nominal_specify=off  T_nominal_value=1  T_nominal_unit=K
  Constant : Constant  Value=273.15
  Convective Heat Transfer : fl_lib/Thermal/Thermal Elements/Convective Heat Transfer  thermal_type=foundation.enum.constant_variable.constant  area=10 m^2  heat_tr_coeff=20 W/(m^2 * K)  min_heat_tr_coeff=1e-3 W/(K*m^2)  T_specify=off  T_priority=None  T=0 K  T_nominal_specify=off  T_nominal_value=1  T_nominal_unit=K  Q_specify=off  Q_priority=None  Q=0 W  Q_nominal_specify=off  Q_nominal_value=1  Q_nominal_unit=W
  Convective Heat Transfer1 : fl_lib/Thermal/Thermal Elements/Convective Heat Transfer  thermal_type=foundation.enum.constant_variable.constant  area=10 m^2  heat_tr_coeff=200 W/(m^2 * K)  min_heat_tr_coeff=1e-3 W/(K*m^2)  T_specify=off  T_priority=None  T=0 K  T_nominal_specify=off  T_nominal_value=1  T_nominal_unit=K  Q_specify=off  Q_priority=None  Q=0 W  Q_nominal_specify=off  Q_nominal_value=1  Q_nominal_unit=W
  PS Terminator : fl_lib/Physical Signals/Sinks/PS Terminator
  PS Terminator1 : fl_lib/Physical Signals/Sinks/PS Terminator
  PS Terminator2 : fl_lib/Physical Signals/Sinks/PS Terminator
  PS-Simulink Converter : nesl_utility/PS-Simulink Converter  PhysicalDomain=network_engine_domain  SubClassName=ps_output  LeftPortType=input  RightPortType=output  PseudoPeriodic=off  Frequencies=[]  VectorFormat=1-D array  Unit=K  AffineConversion=off
  Reservoir (G) : fl_lib/Gas/Elements/Reservoir (G)  pressure_spec=1  reservoir_pressure=0.101325 MPa  reservoir_temperature=25 degC  area_A=0.001 m^2
  Sensor P T : fl_lib/Thermal Liquid/Sensors/Pressure & Temperature Sensor (TL)  reference=foundation.enum.MeasurementReference.difference  pressure=true  pressure_spec=foundation.enum.PressureMeasementSpec.Absolute  temperature=true
      settings: InternalSimscapePortConfiguration="{\"Bottom\":[{\"id\":\"T\",\"label\":\"T\",\"type\":\"output\"}],\"Left\":[{\"id\":\"A\",\"label\":\"A\",\"type\":\"foundation.thermal_liquid.thermal_liquid\"}],\"Right\":[{\"id\":\"B\",\"label\":\"B\",\"type\":\"foundation.thermal_liquid.thermal_liquid\"},{\"id\":\"P\",\"label\":\"P\",\"type\":\"output\"}],\"Top\":[]}"
  Sum : Sum  Inputs=|+-
  Tank : SimscapeFluids_lib/Thermal Liquid/Tanks & Accumulators/Tank (G-TL)  num_inlet=2  volume_total=1 m^3  volume_spec=1  tank_area=0.005 m^2  level_TLU=[0, 3, 5] m  volume_TLU=[0, 4, 6] m^3  inlet_areas_A1B1=[.01, .01] m^2  inlet_height_A2=0.1 m  inlet_area_A2=0.01 m^2  inlet_heights_A2B2=[.01, 0.01] m  inlet_areas_A2B2=[0.1^2/4*pi, 0.1^2/4*pi] m^2  inlet_heights_A2B2C2=[.1, .05, 0] m  inlet_areas_A2B2C2=[.01, .01, .01] m^2  inlet_heights_A2B2C2D2=0.1 * ones(1, 4) m  inlet_areas_A2B2C2D2=0.01 * ones(1, 4) m^2  inlet_heights_A2B2C2D2E2=0.1 * ones(1, 5) m  inlet_areas_A2B2C2D2E2=0.01 * ones(1, 5) m^2  inlet_heights_A2B2C2D2E2F2=0.1 * ones(1, 6) m  inlet_areas_A2B2C2D2E2F2=0.01 * ones(1, 6) m^2  capacity_check=0  max_liquid_capacity=1 m^3  g=9.81 m/s^2  level_specify=on  level_priority=High  level=0.1 m  level_nominal_specify=off  level_nominal_value=1  level_nominal_unit=m  volume_liquid_specify=off  volume_liquid_priority=None  volume_liquid=5 m^3  volume_liquid_nominal_specify=off  volume_liquid_nominal_value=1  volume_liquid_nominal_unit=m^3  mass_liquid_specify=off  mass_liquid_priority=None  mass_liquid=5e+3 kg  mass_liquid_nominal_specify=off  mass_liquid_nominal_value=1  mass_liquid_nominal_unit=kg  T_liquid_specify=on  T_liquid_priority=High  T_liquid=278 K  T_liquid_nominal_specify=off  T_liquid_nominal_value=1  T_liquid_nominal_unit=K  p_gas_specify=off  p_gas_priority=High  p_gas=0.101325 MPa  p_gas_nominal_specify=off  p_gas_nominal_value=1  p_gas_nominal_unit=MPa  T_gas_specify=on  T_gas_priority=High  T_gas=278 K  T_gas_nominal_specify=off  T_gas_nominal_value=1  T_gas_nominal_unit=K  rho_gas_specify=off  rho_gas_priority=None  rho_gas=1.2 kg/m^3  rho_gas_nominal_specify=off  rho_gas_nominal_value=1  rho_gas_nominal_unit=kg/m^3
      settings: InternalSimscapePortConfiguration="{\"Bottom\":[],\"Left\":[{\"id\":\"A1\",\"label\":\"A1\",\"type\":\"foundation.gas.gas\"},{\"id\":\"B1\",\"label\":\"B1\",\"type\":\"foundation.gas.gas\"},{\"id\":\"A2\",\"label\":\"A2\",\"type\":\"foundation.thermal_liquid.thermal_liquid\"},{\"id\":\"B2\",\"label\":\"B2\",\"type\":\"foundation.thermal_liquid.thermal_liquid\"}],\"Right\":[{\"id\":\"H1\",\"label\":\"H1\",\"type\":\"foundation.thermal.thermal\"},{\"id\":\"H2\",\"label\":\"H2\",\"type\":\"foundation.thermal.thermal\"}],\"Top\":[{\"id\":\"V_out\",\"label\":\"V\",\"type\":\"output\"},{\"id\":\"L_out\",\"label\":\"L\",\"type\":\"output\"}]}"
  B : PMIOPort  Side=Left
  HGas : PMIOPort  Port=2  Side=Left
  A : PMIOPort  Port=3  Side=Right
  HLiq : PMIOPort  Port=4  Side=Left
  T : Outport
  wires:
  PS-Simulink Converter/1 -> Sum/1
  Sum/1 -> T/1
  Constant/1 -> Sum/2
  connections:
  Convective Heat Transfer1/LConn1 -- Tank/RConn2
  Sensor P T/LConn1 -- B/RConn1 -- Tank/LConn4
  Absolute Reference (TL)/LConn1 -- Sensor P T/RConn1
  Reservoir (G)/LConn1 -- Tank/LConn1
  Tank/LConn3 -- A/RConn1
  Cap (G)/LConn1 -- Tank/LConn2
  Sensor P T/RConn2 -- PS Terminator2/LConn1
  HGas/RConn1 -- Convective Heat Transfer/RConn1
  Convective Heat Transfer/LConn1 -- Tank/RConn1
  HLiq/RConn1 -- Convective Heat Transfer1/RConn1
  PS-Simulink Converter/LConn1 -- Sensor P T/RConn3
  Tank/LConn5 -- PS Terminator/LConn1
  Tank/LConn6 -- PS Terminator1/LConn1

== system Two_Zone_MVDC_PSolver_Thermal/PMM/Control/Torque Control/Control_System/Current_Controllers ==
  Id : Inport
  Iq : Inport  Port=2
  Idq_ref_PU : Inport  Port=3
  Demux : Demux  Outputs=2
  PI_Controller_Id : Subsystem
  PI_Controller_Iq : Subsystem
  Vd_ref : Outport  VectorParamsAs1DForOutWhenUnconnected=off
  Vq_ref : Outport  Port=2  VectorParamsAs1DForOutWhenUnconnected=off
  wires:
  Iq/1 -> PI_Controller_Iq/2(I_fb)
  Id/1 -> PI_Controller_Id/2(I_fb)
  Idq_ref_PU/1 -> Demux/1
  PI_Controller_Id/1(V_ref) -> Vd_ref/1
  PI_Controller_Iq/1(V_ref) -> Vq_ref/1
  Demux/1 -> PI_Controller_Id/1(I_ref)
  Demux/2 -> PI_Controller_Iq/1(I_ref)

== system Two_Zone_MVDC_PSolver_Thermal/PMM/Control/Torque Control/Control_System/PWM Generator (Three-phase, Two-level) ==
  Vabc : Inport
  vdc : Inport  Port=2
  Data Type Conversion : DataTypeConversion  SaturateOnIntegerOverflow=off  RndMeth=Floor
  Data Type Conversion1 : DataTypeConversion  SaturateOnIntegerOverflow=off  RndMeth=Floor
  Gate Signal Generator : Subsystem
  RTabc : RateTransition  Deterministic=off  OutPortSampleTime=RateTransitionOnInput
  RTdc : RateTransition  Deterministic=off  OutPortSampleTime=RateTransitionOnInput
  Switching Time Calculation : MATLAB Function  TreatAsAtomicUnit=on
  avoid division by 0 : Saturate  UpperLimit=inf  LowerLimit=eps
  g : Outport  VectorParamsAs1DForOutWhenUnconnected=off
  ModWave : Outport  Port=2  VectorParamsAs1DForOutWhenUnconnected=off
  wires:
  vdc/1 -> RTdc/1
  Vabc/1 -> RTabc/1
  Switching Time Calculation/1(TgabcON) -> Gate Signal Generator/1(TgabcON)
  Switching Time Calculation/2(TgabcOFF) -> Gate Signal Generator/2(TgabcOFF)
  Gate Signal Generator/1(s) -> Data Type Conversion/1
  Data Type Conversion/1 -> g/1
  Switching Time Calculation/3(ModWave) -> Data Type Conversion1/1
  RTabc/1 -> Switching Time Calculation/1(Vabc)
  RTdc/1 -> avoid division by 0/1
  avoid division by 0/1 -> Switching Time Calculation/2(vdc)
  Data Type Conversion1/1 -> ModWave/1

== system Two_Zone_MVDC_PSolver_Thermal/PMM/Control/Torque Control/Control_System/ab2abc ==
  ab : Inport
  Demux1 : Demux  Outputs=2
  Mux : Mux  Inputs=3
  Sum : Sum  Inputs=--
  abc : Outport
  wires:
  Demux1/1 -> Sum/2, Mux/1
  Mux/1 -> abc/1
  Sum/1 -> Mux/3
  Demux1/2 -> Sum/1, Mux/2
  ab/1 -> Demux1/1
